simulink model "fullSystemModel"  (R2018a)
settings: Solver=ode3  StartTime=0.0  StopTime=1000  FixedStep=1  MinStep=1e-8  RelTol=1e-8
undefined symbols (not defined in the file or in its folder): DiscIntNeverNeededParam
libraries: BupSimulinkLibraries x32, simulink_extras x22, simulink x2, SignalEditorBlockLib x2
(part 3 of 3)

== stateflow chart fullSystemModel/flightController/TargetSelector ==
  state Initialize
    entry:
    updateIndex = 0;
    targetPoint(latitude) = touchdownPoint(latitude);
    targetPoint(longitude) = touchdownPoint(longitude);
    targetPoint(altitude) = touchdownPoint(altitude);
    targetPoint(relief) = touchdownPointRelief;
  state CheckUpdate
  state ValidateRadioPoint
    entry:
    updateIndex = radioUpdateIndex;
    status = validateTarget();
  state ApplyRadioPoint
    entry:
    targetPoint(latitude) = radioPoint(latitude);
    targetPoint(longitude) = radioPoint(longitude);
    targetPoint(altitude) = radioPoint(altitude);
    targetPoint(relief) = radioPointRelief;
  (default) -> Initialize
  Initialize -> CheckUpdate
  CheckUpdate -> ValidateRadioPoint : [updateIndex~= radioUpdateIndex]
  ApplyRadioPoint -> CheckUpdate
  ValidateRadioPoint -> CheckUpdate [order 2]
  ValidateRadioPoint -> ApplyRadioPoint [order 1] : [status == true]
  data: result function_output boolean size=1; touchdownPoint input double size=3; radioPoint input double size=3; currentPoint input double size=3; targetPoint output double size=4 =[0;0;0;0]; updateIndex local uint8 size=1; radioUpdateIndex input uint8 size=1; latitude constant int8 =1; longitude constant int8 =1; altitude constant int8 =2; verticalVelocity input double size=1; currentCourse input double size=1; status local boolean size=1; airSpeed input double size=1; windForce input double size=1; windCourse input double size=1
  function result = validateTarget:
    | %%%%%%%%%%%%%%%%%%%%%%%%%%%%%%%%%%%%%%%%%%%%%%%%%%%%%%%%%%%%%%%%%%%%%%%%%%%
    | % 
    | %%%%%%%%%%%%%%%%%%%%%%%%%%%%%%%%%%%%%%%%%%%%%%%%%%%%%%%%%%%%%%%%%%%%%%%%%%%
    | function result = validateTarget
    |     %% Определим курс до цели
    |     course = Azimut(radioPoint, currentPoint)
    |     %% Вычислим расстояние с помощью функции DistanceCalculator()
    |     distance = DistanceCalculator(currentPoint, radioPoint);
    |     %% Вычислим скорость по ветру в направлении новой цели
    |     horizontalSpeed = sqrt( airSpeed^2 + windForce^2 - 2*airSpeed*windForce*cos(course-windCourse));
    |     
    |     %% Вычисляем время необходимое для преодоления расстояния до TDP и до посадки
    |     timeHorizontal = distance/horizontalSpeed;
    |     timeVertical = (currentPoint(altitude) - (radioPoint(altitude) + double(radioPoint(relief))))/verticalVelocity;
    |     %% Определяем поправку по времени необходимому на разворот
    |     % Угол разворота
    |     angle = ControlDemode(course - currentCourse);
    |     angle = abs(angle/pi*180);
    |     
    |     % Вычисляем поправку как линейную функцию: 
    |     %timeHorizontalCorrection = angle / TurnSpeed;
    | 
    |     % Вычисляем поправку по параболе
    |     timeHorizontalCorrection = 0.0005*angle^2 + 0.06*angle;
    |         
    |     % Нулевая поправка
    |     timeHorizontalCorrection = 0;
    |     
    |     timeHorizontal = timeHorizontal + timeHorizontalCorrection;
    |     %% Сравшиваем время и выносим результат о теоретической 
    |     % доступности точки
    |     if timeHorizontal < timeVertical
    |         result = true;
    |     else
    |         result = false;
    |     end
    | end
